simulink model "example2"  (Simulink 9.3)
settings: Solver=VariableStepAuto  StartTime=0.0  StopTime=10.0  RelTol=1e-3
settings Model: Creator=root  LastModifiedBy=BEAR
settings DataIOCC: SaveFormat=Dataset  SignalLoggingSaveFormat=Dataset
settings OptimizationCC: LifeSpan=auto
settings DebuggingCC: UnderspecifiedInitializationDetection=Simplified  MergeDetectMultiDrivingBlocksExec=error  FcnCallInpInsideContextMsg=error  SFUnexpectedBacktrackingDiag=error  SFNoUnconditionalDefaultTransitionDiag=error  SFExecutionAtInitializationDiag=warning
settings HardwareCC: ProdBitPerPointer=64  ProdBitPerSizeT=64  ProdBitPerPtrDiffT=64  ProdLargestAtomicFloat=Float  ProdIntDivRoundTo=Zero  ProdEndianess=LittleEndian  ProdWordSize=64  ProdHWDeviceType=Intel->x86-64 (Windows64)
settings ModelReferenceCC: PropagateSignalLabelsOutOfModel=on
settings GRTTargetCC: TargetLangStandard=C99 (ISO)  CombineOutputUpdateFcns=on  GRTInterface=off
settings ConfigComp: CovMetricSettings=dwe  CovHtmlReporting=off  CovSaveCumulativeToWorkspaceVar=off  CovSaveSingleToWorkspaceVar=off  CovExternalEMLEnable=on

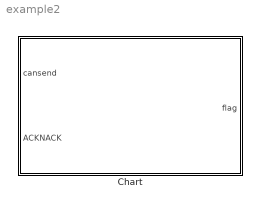
== system example2 ==
  Chart : Stateflow chart  TreatAsAtomicUnit=on

== stateflow chart Chart ==
  state repairing
    during:flag=0
  state waiting
    during:flag=1;
  state must_repair
    during:flag=1;
  repairing -> repairing [order 1] : [cansend]/{re_changes = re_changes - 1}
  must_repair -> repairing [order 1] : after(ResponseDelay,sec)
  must_repair -> must_repair [order 2] : [ACKNACK]/{re_changes = re_changes + 1}
  repairing -> waiting [order 2] : [re_changes==0]
  waiting -> must_repair [order 2] : [re_changes>0]
  (default) -> waiting : {re_changes=0}
  waiting -> waiting [order 1] : [ACKNACK]/{re_changes = re_changes + 1}
  data: flag output double; cansend input double; re_changes local double; ACKNACK input double; ResponseDelay constant double
  events: event local FUNCTION_CALL_EVENT; event1 local FUNCTION_CALL_EVENT
